simulink model "simulink_para_arduino"  (R2021b)
settings: Solver=VariableStepAuto  StartTime=0.0  StopTime=inf  RelTol=1e-3
libraries: instrumentseriallib x2, svdutilitieslib x1, simulink x1
settings Model: Creator=NOTEBOOK  LastModifiedBy=NOTEBOOK

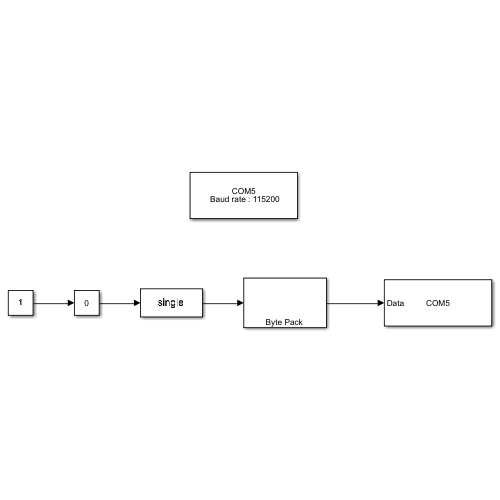
[thumbnail: Simulink's stored preview of the top-level diagram]
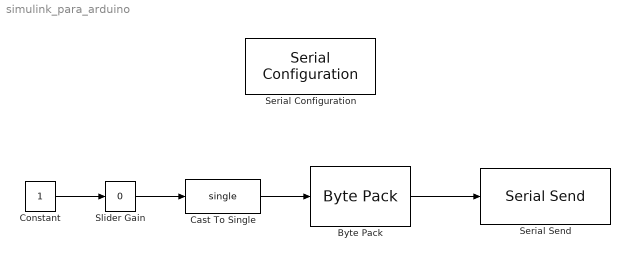
== system simulink_para_arduino ==
  Byte Pack : svdutilitieslib/Byte Pack  maskPackedDataType=uint32  datatypes={'single'}  byteAlign=4  blockPlatform=arduinoert
      settings: SourceProductBaseCode=ANDROID,ARDUINO,ML_ARDUINO,ECCORTEXA,ECCORTEXR,SC_BEAGLEBONE_BLUE,EC_FREEDOM_BOARD,EC_FRDM_K64F,INTEL_BLOCKSET,MICROBIT,NUCLEO,NVIDIA,PX4AUTOPILOTS,RASPPIIO,STMICRODIS,TIC2000,XILINX_BLOCKSET
  Cast To Single : DataTypeConversion  OutDataTypeStr=single
  Constant : Constant  OutDataTypeStr=single
  Serial Configuration : instrumentseriallib/Serial Configuration  Priority=-200000  Port=COM5  ComPort=COM5  BaudRate=115200  DataBits=8  Parity=none  StopBits=1  ByteOrder=little-endian  FlowControl=none  Timeout=10  SimulateUsing=Interpreted execution  BlockInModel=on
  Serial Send : instrumentseriallib/Serial Send  Priority=1  Port=COM5  ComPort=COM5  Header=['A']  Terminator=<none>  CustomTerminator=[]  EnableBlockingMode=on  SimulateUsing=Interpreted execution  BlockInModel=on
  Slider Gain : simulink/Math Operations/Slider Gain  gain=0  low=0  high=180
  wires:
  Constant/1 -> Slider Gain/1
  Cast To Single/1 -> Byte Pack/1
  Byte Pack/1 -> Serial Send/1
  Slider Gain/1 -> Cast To Single/1
